simulink model "Ex10_6_NonlinearPendulum"  (R2023a)
settings: Solver=VariableStepAuto  StartTime=0.0  StopTime=30.0  RelTol=1e-3
settings Model: Creator=Norb  LastModifiedBy=Norb

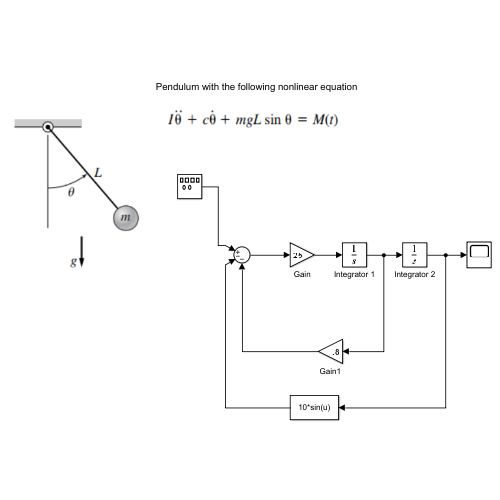
[thumbnail: Simulink's stored preview of the top-level diagram]
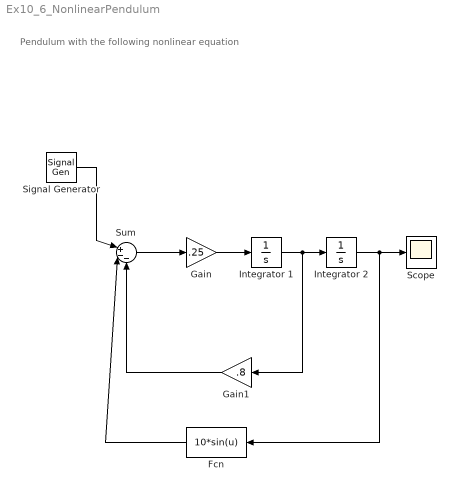
== system Ex10_6_NonlinearPendulum ==
  note: Pendulum with the following nonlinear equation
  Fcn : Fcn  Expr=10*sin(u)
  Gain : Gain  Gain=.25
  Gain1 : Gain  Gain=.8
  Integrator 1 : Integrator
  Integrator 2 : Integrator  InitialCondition=pi/4
  Scope : Scope
  Signal Generator : SignalGenerator  WaveForm=square  Amplitude=3  Frequency=.5
  Sum : Sum  Inputs=|+--
  wires:
  Signal Generator/1 -> Sum/1
  Sum/1 -> Gain/1
  Gain/1 -> Integrator 1/1
  Integrator 1/1 -> Gain1/1, Integrator 2/1
  Integrator 2/1 -> Fcn/1, Scope/1
  Fcn/1 -> Sum/2
  Gain1/1 -> Sum/3
